simulink model "essai_1"  (R2018a)
settings: Solver=VariableStepAuto  StartTime=0.0  StopTime=10.0  RelTol=1e-3
libraries: simulink_extras x3, simulink x2
settings Model: Creator=bobau  LastModifiedBy=bobau

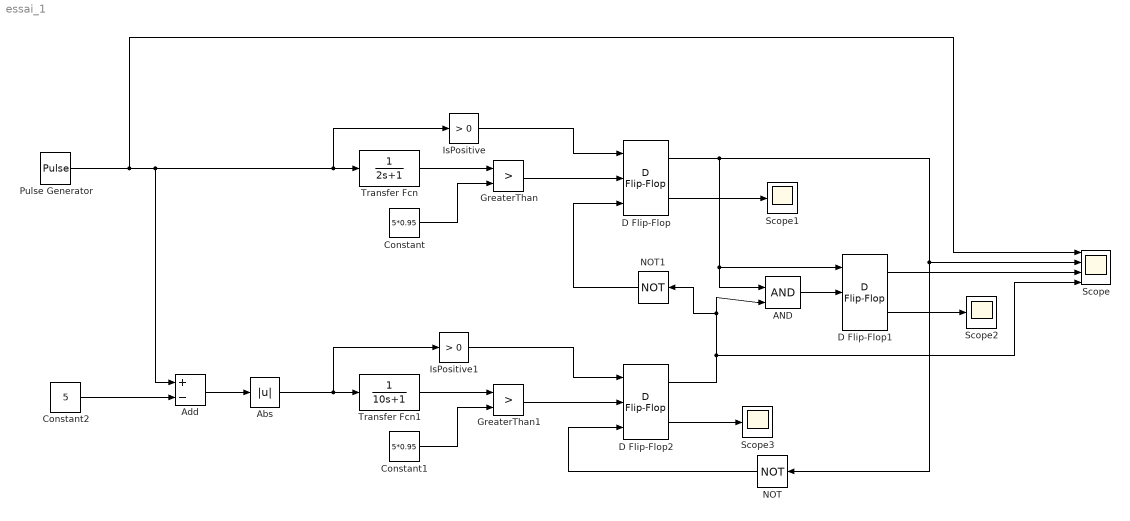
== system essai_1 ==
  AND : Logic  IconShape=distinctive  AllPortsSameDT=off  OutDataTypeStr=boolean
  Abs : Abs
  Add : Sum  Inputs=+-
  Constant : Constant  Value=5*0.95
  Constant1 : Constant  Value=5*0.95
  Constant2 : Constant  Value=5
  D Flip-Flop : simulink_extras/Flip Flops/D Flip-Flop
      settings: SourceProductName=Simulink
  D Flip-Flop1 : simulink_extras/Flip Flops/D Flip-Flop
      settings: SourceProductName=Simulink
  D Flip-Flop2 : simulink_extras/Flip Flops/D Flip-Flop
      settings: SourceProductName=Simulink
  GreaterThan : RelationalOperator  Operator=>  OutDataTypeStr=boolean  RndMeth=Simplest
  GreaterThan1 : RelationalOperator  Operator=>  OutDataTypeStr=boolean  RndMeth=Simplest
  IsPositive : simulink/Logic and Bit Operations/Compare To Zero  relop=>  OutDataTypeStr=boolean
  IsPositive1 : simulink/Logic and Bit Operations/Compare To Zero  relop=>  OutDataTypeStr=boolean
  NOT : Logic  Operator=NOT  IconShape=distinctive  AllPortsSameDT=off  OutDataTypeStr=boolean
  NOT1 : Logic  Operator=NOT  IconShape=distinctive  AllPortsSameDT=off  OutDataTypeStr=boolean
  Pulse Generator : DiscretePulseGenerator  PulseType=Time based  Amplitude=5  Period=10  PulseWidth=5
  Scope : Scope  NumInputPorts=4
  Scope1 : Scope
  Scope2 : Scope
  Scope3 : Scope
  Transfer Fcn : TransferFcn  Denominator=[2 1]
  Transfer Fcn1 : TransferFcn  Denominator=[10 1]
  wires:
  Transfer Fcn/1 -> GreaterThan/1
  Constant/1 -> GreaterThan/2
  Pulse Generator/1 -> Scope/1, Add/1, IsPositive/1, Transfer Fcn/1
  GreaterThan/1 -> D Flip-Flop/2
  D Flip-Flop/1 -> Scope/2, NOT/1, AND/1, D Flip-Flop1/1
  AND/1 -> D Flip-Flop1/2
  GreaterThan1/1 -> D Flip-Flop2/2
  Abs/1 -> Transfer Fcn1/1, IsPositive1/1
  Constant1/1 -> GreaterThan1/2
  Transfer Fcn1/1 -> GreaterThan1/1
  Constant2/1 -> Add/2
  Add/1 -> Abs/1
  NOT/1 -> D Flip-Flop2/3
  NOT1/1 -> D Flip-Flop/3
  D Flip-Flop2/1 -> Scope/4, NOT1/1, AND/2
  D Flip-Flop1/1 -> Scope/3
  D Flip-Flop/2 -> Scope1/1
  D Flip-Flop1/2 -> Scope2/1
  D Flip-Flop2/2 -> Scope3/1
  IsPositive/1 -> D Flip-Flop/1
  IsPositive1/1 -> D Flip-Flop2/1
